simulink model "Project2_egyenlet"  (R2024b)
settings: Solver=VariableStepAuto  StartTime=0.0  StopTime=10.0  RelTol=1e-3
values from neighbouring files (symbols this model uses):
  A = 3    [Project2_egyenlet_run.m]
  F = 2    [Project2_egyenlet_run.m]
  Ti = 0.5    [Project2_egyenlet_run.m]
settings Model: Creator=szala  LastModifiedBy=szala

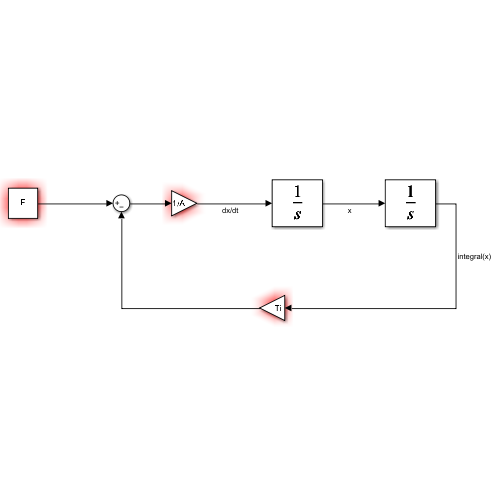
[thumbnail: Simulink's stored preview of the top-level diagram]
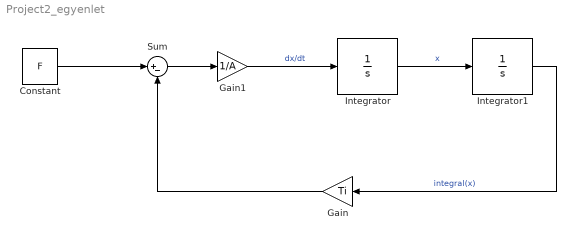
== system Project2_egyenlet ==
  Constant : Constant  Value=F
  Gain : Gain  Gain=Ti
  Gain1 : Gain  Gain=1/A
  Integrator : Integrator
  Integrator1 : Integrator
  Sum : Sum  Inputs=|+-
  wires:
  Integrator/1 -> Integrator1/1  "x"
  Gain1/1 -> Integrator/1  "dx/dt"
  Integrator1/1 -> Gain/1  "integral(x)"
  Constant/1 -> Sum/1
  Gain/1 -> Sum/2
  Sum/1 -> Gain1/1
